simulink model "TPTC_Vehicle_dynamics_pedal2torque_NeglectSOC"  (R2026a)
settings: Solver=ode23tb  StopTime=40
model workspace (MAT data in the model file):
  BattChrgMax = -500000
  BattDischrgMax = 500000
  ChrgLmt_bpt = [1 1 1 1 1 1 1 1 0.7 0.35 0]
  DischrgLmt_bpt = [0 0.35 0.7 1 1 1 1 1 1 1 1]
  SOC_bpt = [0 10 20 30 40 50 60 70 80 90 100]
  motorMaxTorqueNm = [500 500 500 500 500 500 416.666666667 357.142857143 312.5 277.777777778 250 227.272727273 ... (16 elements, 1x16)]
  motorSpeedRadPs = [0 40 80 120 160 200 240 280 320 360 400 440 ... (16 elements, 1x16)]
values from neighbouring files (symbols this model uses):
  alpha_thr = Simulink.Parameter(300)    [init_MCU_ASR_params_only.m]
  eta_drv = Simulink.Parameter(0.95)    [init_MCU_ASR_params_only.m]
  gear_ratio_F = Simulink.Parameter(10.91)    [init_MCU_ASR_params_only.m]
  gear_ratio_R = Simulink.Parameter(11.62)    [init_MCU_ASR_params_only.m]
  J_axle = Simulink.Parameter(2*I_tire)    [init_MCU_ASR_params_only.m]
  Kd_damp = Simulink.Parameter(0.025)    [init_MCU_ASR_params_only.m]
  R_tire = Simulink.Parameter(r)    [init_MCU_ASR_params_only.m]
  T_active = Simulink.Parameter(15)    [init_MCU_ASR_params_only.m]
  T_damp_lim = Simulink.Parameter(18)    [init_MCU_ASR_params_only.m]
  tau_lpf_damp = Simulink.Parameter(0.060)    [init_MCU_ASR_params_only.m]
  Tlim_down_rate = Simulink.Parameter(2000)    [init_MCU_ASR_params_only.m]
  Tlim_up_rate = Simulink.Parameter(120)    [init_MCU_ASR_params_only.m]
  Tlim_warn_rate = Simulink.Parameter(600)    [init_MCU_ASR_params_only.m]
  Tmax_mot = Simulink.Parameter(Tn_motor)    [init_MCU_ASR_params_only.m]
  Ts_asr = Simulink.Parameter(0.001)    [init_MCU_ASR_params_only.m]
undefined symbols (not defined in the file or in its folder): dspblkCoreblockFVToolHelper, gcbh, gear_ratio
libraries: autolibsharedcoupling x8, simulink x3, autolibshareddiff x2, autolibmappedmotor x2, slpidlib x1, autolibdatasheetbattery x1, sim3dlib x1, sim3dautolib x1, vehdynlibsteering x1
(part 2 of 4)

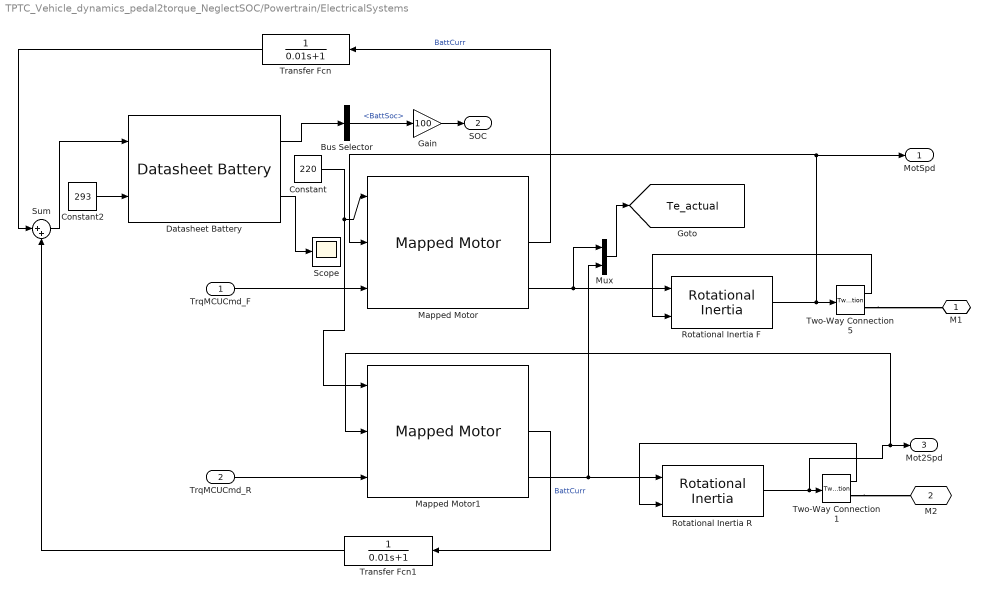
== system TPTC_Vehicle_dynamics_pedal2torque_NeglectSOC/Powertrain/ElectricalSystems ==
  TrqMCUCmd_F : Inport
  TrqMCUCmd_R : Inport  Port=2
  Bus Selector : BusSelector  OutputSignals=BattSoc
  Constant : Constant  Value=220
  Constant2 : Constant  Value=293
  Datasheet Battery : autolibdatasheetbattery/Datasheet Battery  CapacityCtrl=Parameter  OutputVlt=Unfiltered  BattChargeMax=100  Em=[2.8 3.228 3.284 3.361 3.408 3.427 3.472 3.477 3.493 3.504 3.516 3.528 3.537 3.545 3.555 3.561 3.566 3.576 3.587 3.589 3.594 3.6 3.608 3.61 3.616 3.619 3.626 3.632 3.637 3.64 3.645 3.646 3.652 3.655 3.658 3.661 3.664 3.668 3.673 3.678 3.68 3.681 3.686 3.692 3.699 3.702 3.705 3.71 3.717 3.723 3.728 3.733 3.735 3.742 3.749 3.755 3.761 3.768 3.773 3.78 3.791 3.798 3.798 3.814 3.818 3.825 3.841 3.846 3.855 3.863 3.877 3.885 3.894 3.907 3.919 3.926 3.935 3.944 3.954 3.964 3.974 3.988 3.998 4.014 4.029 4.034 4.047 4.065 4.074 4.086 4.097 4.131 4.126 4.138 4.15 4.18 4.174 4.187 4.207 4.231 4.221]  SOCEmBp=[0 0.01 0.02 0.03 0.04 0.05 0.06 0.07 0.08 0.09 0.1 0.11 0.12 0.13 0.14 0.15 0.16 0.17 0.18 0.19 0.2 0.21 0.22 0.23 0.24 0.25 0.26 0.27 0.28 0.29 0.3 0.31 0.32 0.33 0.34 0.35 0.36 0.37 0.38 0.39 0.4 0.41 0.42 0.43 0.44 0.45 0.46 0.47 0.48 0.49 0.5 0.51 0.52 0.53 0.54 0.55 0.56 0.57 0.58 0.59 0.6 0.61 0.62 0.63 0.64 0.65 0.66 0.67 0.68 0.69 0.7 0.71 0.72 0.73 0.74 0.75 0.76 0.77 0.78 0.79 0.8 0.81 0.82 0.83 0.84 0.85 0.86 0.87 0.88 0.89 0.9 0.91 0.92 0.93 0.94 0.95 0.96 0.97 0.98 0.99 1]  RInt=[0.008846 0.009319 0.009027 0.00847 0.01032 0.01314;0.006389 0.006554 0.005553 0.005525 0.006043 0.007805;0.004364 0.004101 0.00406 0.003452 0.003846 0.004517;0.002031 0.002563 0.002532 0.00246 0.002716 0.003047;0.001443 0.001825 0.001795 0.001778 0.001924 0.002234;0.0005603 0.0007192 0.0006887 0.0007557 0.0007355 0.001014;0.001028 0.001338 0.001 0.001536 0.001546 0.002789]  BattTempBp=[243.1 253.1 263.1 273.1 283.1 298.1 313.1]  SOCRintBp=[0 0.2 0.4 0.6 0.8 1]  Ns=30  Np=2  BattCapInit=60  Tc=1/1000  Vinit=4.221  RefBlkName='autolibdatasheetbattery/Datasheet Battery'
  Gain : Gain  Gain=100
  Mapped Motor : autolibmappedmotor/Mapped Motor  w_Tmax_bp_ext=w_Tmax_bp  Tmax_w_V_ext=Tmax_w_V  w_Tmin_bp_ext=w_Tmin_bp  Tmin_w_V_ext=Tmin_w_V  port_config=Speed  param_by=Tabulated torque-speed envelope  w_t=motorSpeedRadPs  T_t=motorMaxTorqueNm  torque_max=.1  power_max=30  SpreadsheetTqLimitsFileName=MotorCalibrationImportData.xlsx  Tmax_w_V=[0.09 0.09 0.09;0.08 0.08 0.08;0.07 0.07 0.07;0 0 0]  w_Tmax_bp=[ 0 375 750 800 ]  V_Tmax_bp=[500 750 900]  Tmin_w_V=[-0.09 -0.09 -0.09;-0.08 -0.08 -0.08;-0.07 -0.07 -0.07;0 0 0]  w_Tmin_bp=[ 0 375 750 800 ]  V_Tmin_bp=[500 750 900]  Tc=0.02  param_loss=Single efficiency measurement  SpreadsheetLossFileName=MotorCalibrationImportData.xlsx  SpreadsheetEffFileName=MotorCalibrationImportData.xlsx  eff=100  w_eff=375  T_eff=0.08  Piron=0  Pbase=0  w_eff_bp=[-8000 -4000 0 4000 8000]  T_eff_bp=[0 0.03 0.06 0.09]  Temp_eff_bp=[233.15 293.15 373.15]  V_eff_bp=[500 700 900]  losses_table=[1.49 1.67 2.21 3.10; 0.42 0.69 1.14 2.03; 0.06 0.24 0.78 1.68; 0.42 0.69 1.14 2.03; 1.49 1.67 2.21 3.10]  losses_table_3d=cat(3,1.05*[1.49 1.67 2.21 3.10; 0.42 0.69 1.14 2.03; 0.06 0.24 0.78 1.68; 0.42 0.69 1.14 2.03; 1.49 1.67 2.21 3.10],[1.49 1.67 2.21 3.10; 0.42 0.69 1.14 2.03; 0.06 0.24 0.78 1.68; 0.42 0.69 1.14 2.03; 1.49 1.67 2.21 3.10],1.03*[1.49 1.67 2.21 3.10; 0.42 0.69 1.14 2.03; 0.06 0.24 0.78 1.68; 0.42 0.69 1.14 2.03; 1.49 1.67 2.21 3.10])  losses_table_4d=cat(4,cat(3,[1.5645 0.441 0.063 0.441 1.5645;1.7535 0.7245 0.252 0.7245 1.7535;2.3205 1.197 0.819 1.197 2.3205;3.255 2.1315 1.764 2.1315 3.255],[1.5645 0.441 0.063 0.441 1.5645;1.7535 0.7245 0.252 0.7245 1.7535;2.3205 1.197 0.819 1.197 2.3205;3.255 2.1315 1.764 2.1315 3.255],[1.5645 0.441 0.063 0.441 1.5645;1.7535 0.7245 0.252 0.7245 1.7535;2.3205 1.197 0.819 1.197 2.3205;3.255 2.1315 1.764 2.1315 3.255]),cat(3,[1.49 0.42 0.06 0.42 1.49;1.67 0.69 0.24 0.69 1.67;2.21 1.14 0.78 1.14 2.21;3.1 2.03 1.68 2.03 3.1],[1.49 0.42 0.06 0.42 1.49;1.67 0.69 0.24 0.69 1.67;2.21 1.14 0.78 1.14 2.21;3.1 2.03 1.68 2.03 3.1],[1.49 0.42 0.06 0.42 1.49;1.67 0.69 0.24 0.69 1.67;2.21 1.14 0.78 1.14 2.21;3.1 2.03 1.68 2.03 3.1]),cat(3,[1.5347 0.4326 0.0618 0.4326 1.5347;1.7201 0.7107 0.2472 0.7107 1.7201;2.2763 1.1742 0.8034 1.1742 2.2763;3.193 2.0909 1.7304 2.0909 3.193],[1.5347 0.4326 0.0618 0.4326 1.5347;1.7201 0.7107 0.2472 0.7107 1.7201;2.2763 1.1742 0.8034 1.1742 2.2763;3.193 2.0909 1.7304 2.0909 3.193],[1.5347 0.4326 0.0618 0.4326 1.5347;1.7201 0.7107 0.2472 0.7107 1.7201;2.2763 1.1742 0.8034 1.1742 2.2763;3.193 2.0909 1.7304 2.0909 3.193]))  efficiency_table=[95 95 95 95; 95 95 95 95; 95 95 95 95; 95 95 95 95; 95 95 95 95]  efficiency_table_3d=cat(3,90*ones(5,4),95*ones(5,4),92*ones(5,4))  efficiency_table_4d=cat(4,cat(3,90*ones(5,4)',90*ones(5,4)',90*ones(5,4)'),cat(3,95*ones(5,4)',95*ones(5,4)',95*ones(5,4)'),cat(3,92*ones(5,4)',92*ones(5,4)',92*ones(5,4)'))  J=5e-6  b=1e-5  omega_o=0  T_t_extended=[166.666666666667 178.571428571429 192.307692307692 208.333333333333 227.272727272727 250 277.777777777778 312.5 357.142857142857 416.666666666667 500 500 500 500 500 500 500 500 500 500 500 416.666666666667 357.142857142857 312.5 277.777777777778 250 227.272727272727 208.333333333333 192.307692307692 178.571428571429 166.666666666667]  w_t_extended=[-600 -560 -520 -480 -440 -400 -360 -320 -280 -240 -200 -160 -120 -80 -40 0 40 80 120 160 200 240 280 320 360 400 440 480 520 560 600]  KLossIron=0  KLossCopper=0  x_w_eff_vec=[-8000 -4000 0 4000 8000]  x_T_eff_vec=[-0.09 -0.06 -0.03 0 0.03 0.06 0.09]  x_tmp_eff_vec=[233.15 293.15 373.15]  x_V_eff_vec=[500 700 900]  x_losses_mat=[3.1 2.21 1.67 1.49 1.67 2.21 3.1;2.03 1.14 0.69 0.42 0.69 1.14 2.03;1.68 0.78 0.24 0.06 0.24 0.78 1.68;2.03 1.14 0.69 0.42 0.69 1.14 2.03;3.1 2.21 1.67 1.49 1.67 2.21 3.1]  x_losses_mat_3d=cat(3,[3.255 2.3205 1.7535 1.5645 1.7535 2.3205 3.255;2.1315 1.197 0.7245 0.441 0.7245 1.197 2.1315;1.764 0.819 0.252 0.063 0.252 0.819 1.764;2.1315 1.197 0.7245 0.441 0.7245 1.197 2.1315;3.255 2.3205 1.7535 1.5645 1.7535 2.3205 3.255],[3.1 2.21 1.67 1.49 1.67 2.21 3.1;2.03 1.14 0.69 0.42 0.69 1.14 2.03;1.68 0.78 0.24 0.06 0.24 0.78 1.68;2.03 1.14 0.69 0.42 0.69 1.14 2.03;3.1 2.21 1.67 1.49 1.67 2.21 3.1],[3.193 2.2763 1.7201 1.5347 1.7201 2.2763 3.193;2.0909 1.1742 0.7107 0.4326 0.7107 1.1742 2.0909;1.7304 0.8034 0.2472 0.0618 0.2472 0.8034 1.7304;2.0909 1.1742 0.7107 0.4326 0.7107 1.1742 2.0909;3.193 2.2763 1.7201 1.5347 1.7201 2.2763 3.193])  x_losses_mat_4d=cat(4,cat(3,[1.5645 0.441 0.063 0.441 1.5645;1.7535 0.7245 0.252 0.7245 1.7535;2.3205 1.197 0.819 1.197 2.3205;3.255 2.1315 1.764 2.1315 3.255],[1.5645 0.441 0.063 0.441 1.5645;1.7535 0.7245 0.252 0.7245 1.7535;2.3205 1.197 0.819 1.197 2.3205;3.255 2.1315 1.764 2.1315 3.255],[1.5645 0.441 0.063 0.441 1.5645;1.7535 0.7245 0.252 0.7245 1.7535;2.3205 1.197 0.819 1.197 2.3205;3.255 2.1315 1.764 2.1315 3.255]),cat(3,[1.49 0.42 0.06 0.42 1.49;1.67 0.69 0.24 0.69 1.67;2.21 1.14 0.78 1.14 2.21;3.1 2.03 1.68 2.03 3.1],[1.49 0.42 0.06 0.42 1.49;1.67 0.69 0.24 0.69 1.67;2.21 1.14 0.78 1.14 2.21;3.1 2.03 1.68 2.03 3.1],[1.49 0.42 0.06 0.42 1.49;1.67 0.69 0.24 0.69 1.67;2.21 1.14 0.78 1.14 2.21;3.1 2.03 1.68 2.03 3.1]),cat(3,[1.5347 0.4326 0.0618 0.4326 1.5347;1.7201 0.7107 0.2472 0.7107 1.7201;2.2763 1.1742 0.8034 1.1742 2.2763;3.193 2.0909 1.7304 2.0909 3.193],[1.5347 0.4326 0.0618 0.4326 1.5347;1.7201 0.7107 0.2472 0.7107 1.7201;2.2763 1.1742 0.8034 1.1742 2.2763;3.193 2.0909 1.7304 2.0909 3.193],[1.5347 0.4326 0.0618 0.4326 1.5347;1.7201 0.7107 0.2472 0.7107 1.7201;2.2763 1.1742 0.8034 1.1742 2.2763;3.193 2.0909 1.7304 2.0909 3.193]))  CalLossMapData={}  CalLossWithTempMapData={}  aMode=aMode  RefBlkName='autolibmappedmotor/Mapped Motor'
  Mapped Motor1 : autolibmappedmotor/Mapped Motor  w_Tmax_bp_ext=w_Tmax_bp  Tmax_w_V_ext=Tmax_w_V  w_Tmin_bp_ext=w_Tmin_bp  Tmin_w_V_ext=Tmin_w_V  port_config=Speed  param_by=Tabulated torque-speed envelope  w_t=motorSpeedRadPs  T_t=motorMaxTorqueNm  torque_max=.1  power_max=30  SpreadsheetTqLimitsFileName=MotorCalibrationImportData.xlsx  Tmax_w_V=[0.09 0.09 0.09;0.08 0.08 0.08;0.07 0.07 0.07;0 0 0]  w_Tmax_bp=[ 0 375 750 800 ]  V_Tmax_bp=[500 750 900]  Tmin_w_V=[-0.09 -0.09 -0.09;-0.08 -0.08 -0.08;-0.07 -0.07 -0.07;0 0 0]  w_Tmin_bp=[ 0 375 750 800 ]  V_Tmin_bp=[500 750 900]  Tc=0.02  param_loss=Single efficiency measurement  SpreadsheetLossFileName=MotorCalibrationImportData.xlsx  SpreadsheetEffFileName=MotorCalibrationImportData.xlsx  eff=100  w_eff=375  T_eff=0.08  Piron=0  Pbase=0  w_eff_bp=[-8000 -4000 0 4000 8000]  T_eff_bp=[0 0.03 0.06 0.09]  Temp_eff_bp=[233.15 293.15 373.15]  V_eff_bp=[500 700 900]  losses_table=[1.49 1.67 2.21 3.10; 0.42 0.69 1.14 2.03; 0.06 0.24 0.78 1.68; 0.42 0.69 1.14 2.03; 1.49 1.67 2.21 3.10]  losses_table_3d=cat(3,1.05*[1.49 1.67 2.21 3.10; 0.42 0.69 1.14 2.03; 0.06 0.24 0.78 1.68; 0.42 0.69 1.14 2.03; 1.49 1.67 2.21 3.10],[1.49 1.67 2.21 3.10; 0.42 0.69 1.14 2.03; 0.06 0.24 0.78 1.68; 0.42 0.69 1.14 2.03; 1.49 1.67 2.21 3.10],1.03*[1.49 1.67 2.21 3.10; 0.42 0.69 1.14 2.03; 0.06 0.24 0.78 1.68; 0.42 0.69 1.14 2.03; 1.49 1.67 2.21 3.10])  losses_table_4d=cat(4,cat(3,[1.5645 0.441 0.063 0.441 1.5645;1.7535 0.7245 0.252 0.7245 1.7535;2.3205 1.197 0.819 1.197 2.3205;3.255 2.1315 1.764 2.1315 3.255],[1.5645 0.441 0.063 0.441 1.5645;1.7535 0.7245 0.252 0.7245 1.7535;2.3205 1.197 0.819 1.197 2.3205;3.255 2.1315 1.764 2.1315 3.255],[1.5645 0.441 0.063 0.441 1.5645;1.7535 0.7245 0.252 0.7245 1.7535;2.3205 1.197 0.819 1.197 2.3205;3.255 2.1315 1.764 2.1315 3.255]),cat(3,[1.49 0.42 0.06 0.42 1.49;1.67 0.69 0.24 0.69 1.67;2.21 1.14 0.78 1.14 2.21;3.1 2.03 1.68 2.03 3.1],[1.49 0.42 0.06 0.42 1.49;1.67 0.69 0.24 0.69 1.67;2.21 1.14 0.78 1.14 2.21;3.1 2.03 1.68 2.03 3.1],[1.49 0.42 0.06 0.42 1.49;1.67 0.69 0.24 0.69 1.67;2.21 1.14 0.78 1.14 2.21;3.1 2.03 1.68 2.03 3.1]),cat(3,[1.5347 0.4326 0.0618 0.4326 1.5347;1.7201 0.7107 0.2472 0.7107 1.7201;2.2763 1.1742 0.8034 1.1742 2.2763;3.193 2.0909 1.7304 2.0909 3.193],[1.5347 0.4326 0.0618 0.4326 1.5347;1.7201 0.7107 0.2472 0.7107 1.7201;2.2763 1.1742 0.8034 1.1742 2.2763;3.193 2.0909 1.7304 2.0909 3.193],[1.5347 0.4326 0.0618 0.4326 1.5347;1.7201 0.7107 0.2472 0.7107 1.7201;2.2763 1.1742 0.8034 1.1742 2.2763;3.193 2.0909 1.7304 2.0909 3.193]))  efficiency_table=[95 95 95 95; 95 95 95 95; 95 95 95 95; 95 95 95 95; 95 95 95 95]  efficiency_table_3d=cat(3,90*ones(5,4),95*ones(5,4),92*ones(5,4))  efficiency_table_4d=cat(4,cat(3,90*ones(5,4)',90*ones(5,4)',90*ones(5,4)'),cat(3,95*ones(5,4)',95*ones(5,4)',95*ones(5,4)'),cat(3,92*ones(5,4)',92*ones(5,4)',92*ones(5,4)'))  J=5e-6  b=1e-5  omega_o=0  T_t_extended=[166.666666666667 178.571428571429 192.307692307692 208.333333333333 227.272727272727 250 277.777777777778 312.5 357.142857142857 416.666666666667 500 500 500 500 500 500 500 500 500 500 500 416.666666666667 357.142857142857 312.5 277.777777777778 250 227.272727272727 208.333333333333 192.307692307692 178.571428571429 166.666666666667]  w_t_extended=[-600 -560 -520 -480 -440 -400 -360 -320 -280 -240 -200 -160 -120 -80 -40 0 40 80 120 160 200 240 280 320 360 400 440 480 520 560 600]  KLossIron=0  KLossCopper=0  x_w_eff_vec=[-8000 -4000 0 4000 8000]  x_T_eff_vec=[-0.09 -0.06 -0.03 0 0.03 0.06 0.09]  x_tmp_eff_vec=[233.15 293.15 373.15]  x_V_eff_vec=[500 700 900]  x_losses_mat=[3.1 2.21 1.67 1.49 1.67 2.21 3.1;2.03 1.14 0.69 0.42 0.69 1.14 2.03;1.68 0.78 0.24 0.06 0.24 0.78 1.68;2.03 1.14 0.69 0.42 0.69 1.14 2.03;3.1 2.21 1.67 1.49 1.67 2.21 3.1]  x_losses_mat_3d=cat(3,[3.255 2.3205 1.7535 1.5645 1.7535 2.3205 3.255;2.1315 1.197 0.7245 0.441 0.7245 1.197 2.1315;1.764 0.819 0.252 0.063 0.252 0.819 1.764;2.1315 1.197 0.7245 0.441 0.7245 1.197 2.1315;3.255 2.3205 1.7535 1.5645 1.7535 2.3205 3.255],[3.1 2.21 1.67 1.49 1.67 2.21 3.1;2.03 1.14 0.69 0.42 0.69 1.14 2.03;1.68 0.78 0.24 0.06 0.24 0.78 1.68;2.03 1.14 0.69 0.42 0.69 1.14 2.03;3.1 2.21 1.67 1.49 1.67 2.21 3.1],[3.193 2.2763 1.7201 1.5347 1.7201 2.2763 3.193;2.0909 1.1742 0.7107 0.4326 0.7107 1.1742 2.0909;1.7304 0.8034 0.2472 0.0618 0.2472 0.8034 1.7304;2.0909 1.1742 0.7107 0.4326 0.7107 1.1742 2.0909;3.193 2.2763 1.7201 1.5347 1.7201 2.2763 3.193])  x_losses_mat_4d=cat(4,cat(3,[1.5645 0.441 0.063 0.441 1.5645;1.7535 0.7245 0.252 0.7245 1.7535;2.3205 1.197 0.819 1.197 2.3205;3.255 2.1315 1.764 2.1315 3.255],[1.5645 0.441 0.063 0.441 1.5645;1.7535 0.7245 0.252 0.7245 1.7535;2.3205 1.197 0.819 1.197 2.3205;3.255 2.1315 1.764 2.1315 3.255],[1.5645 0.441 0.063 0.441 1.5645;1.7535 0.7245 0.252 0.7245 1.7535;2.3205 1.197 0.819 1.197 2.3205;3.255 2.1315 1.764 2.1315 3.255]),cat(3,[1.49 0.42 0.06 0.42 1.49;1.67 0.69 0.24 0.69 1.67;2.21 1.14 0.78 1.14 2.21;3.1 2.03 1.68 2.03 3.1],[1.49 0.42 0.06 0.42 1.49;1.67 0.69 0.24 0.69 1.67;2.21 1.14 0.78 1.14 2.21;3.1 2.03 1.68 2.03 3.1],[1.49 0.42 0.06 0.42 1.49;1.67 0.69 0.24 0.69 1.67;2.21 1.14 0.78 1.14 2.21;3.1 2.03 1.68 2.03 3.1]),cat(3,[1.5347 0.4326 0.0618 0.4326 1.5347;1.7201 0.7107 0.2472 0.7107 1.7201;2.2763 1.1742 0.8034 1.1742 2.2763;3.193 2.0909 1.7304 2.0909 3.193],[1.5347 0.4326 0.0618 0.4326 1.5347;1.7201 0.7107 0.2472 0.7107 1.7201;2.2763 1.1742 0.8034 1.1742 2.2763;3.193 2.0909 1.7304 2.0909 3.193],[1.5347 0.4326 0.0618 0.4326 1.5347;1.7201 0.7107 0.2472 0.7107 1.7201;2.2763 1.1742 0.8034 1.1742 2.2763;3.193 2.0909 1.7304 2.0909 3.193]))  CalLossMapData={}  CalLossWithTempMapData={}  aMode=aMode  RefBlkName='autolibmappedmotor/Mapped Motor'
  Mux : Mux  Inputs=2
  Rotational Inertia F : autolibsharedcoupling/Rotational Inertia  port_config=Simulink  extInfo=off  externJ=off  J=.001  b=.001  omega_o=0  blkID=0  aMode=1
      settings: LibrarySourceBlock=autolibcoupling/Rotational Inertia
  Rotational Inertia R : autolibsharedcoupling/Rotational Inertia  port_config=Simulink  extInfo=off  externJ=off  J=.001  b=.001  omega_o=0  blkID=0  aMode=1
      settings: LibrarySourceBlock=autolibcoupling/Rotational Inertia
  Scope : Scope
      settings: ActiveDisplayYMinimum=56.73874  ActiveDisplayYMaximum=120.06236  DataLoggingVariableName=ScopeData18
  Sum : Sum  Inputs=|++
  Transfer Fcn : TransferFcn  Denominator=[0.01 1]
  Transfer Fcn1 : TransferFcn  Denominator=[0.01 1]
  Two-Way Connection1 : TwoWayConnection
  Two-Way Connection5 : TwoWayConnection
  M1 : PMIOPort  Side=Right
  M2 : PMIOPort  Port=2  Side=Right
  MotSpd : Outport
  SOC : Outport  Port=2
  Mot2Spd : Outport  Port=3
  tag scope: Te_actual=global
  wires:
  Rotational Inertia F/1 -> Mapped Motor/2, MotSpd/1, Two-Way Connection5/1
  Datasheet Battery/2 -> Scope/1
  Mapped Motor/3 -> Mux/1, Rotational Inertia F/1
  TrqMCUCmd_F/1 -> Mapped Motor/3
  Two-Way Connection5/1 -> Rotational Inertia F/2
  Constant2/1 -> Datasheet Battery/2
  Mapped Motor/2 -> Transfer Fcn/1  "BattCurr"
  Datasheet Battery/1 -> Bus Selector/1
  Bus Selector/1 -> Gain/1  "<BattSoc>"
  Gain/1 -> SOC/1
  Rotational Inertia R/1 -> Mapped Motor1/2, Mot2Spd/1, Two-Way Connection1/1
  Mapped Motor1/3 -> Mux/2, Rotational Inertia R/1
  Two-Way Connection1/1 -> Rotational Inertia R/2
  TrqMCUCmd_R/1 -> Mapped Motor1/3
  Mapped Motor1/2 -> Transfer Fcn1/1  "BattCurr"
  Transfer Fcn/1 -> Sum/1
  Transfer Fcn1/1 -> Sum/2
  Sum/1 -> Datasheet Battery/1
  Mux/1 -> [Te_actual]
  Constant/1 -> Mapped Motor1/1, Mapped Motor/1
  connections:
  Two-Way Connection5/RConn1 -- M1/RConn1
  Two-Way Connection1/RConn1 -- M2/RConn1

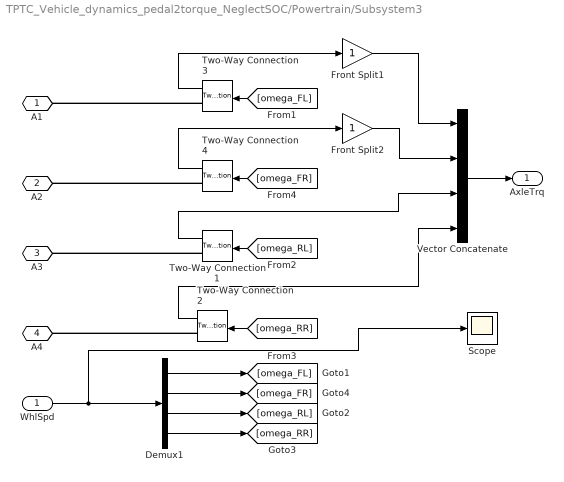
== system TPTC_Vehicle_dynamics_pedal2torque_NeglectSOC/Powertrain/Subsystem3 ==
  WhlSpd : Inport
  Demux1 : Demux
  Front Split1 : Gain
  Front Split2 : Gain
  Scope : Scope
      settings: ActiveDisplayYMinimum=-39.72739  ActiveDisplayYMaximum=357.54646  DataLoggingVariableName=ScopeData19
  Two-Way Connection{1..4} (4 alike) : TwoWayConnection
  Vector Concatenate : Concatenate  NumInputs=4
  A1 : PMIOPort  Side=Left
  A2 : PMIOPort  Port=2  Side=Left
  A3 : PMIOPort  Port=3  Side=Left
  A4 : PMIOPort  Port=4  Side=Left
  AxleTrq : Outport  VectorParamsAs1DForOutWhenUnconnected=off
  wires:
  Two-Way Connection1/1 -> Vector Concatenate/3
  Front Split1/1 -> Vector Concatenate/1
  [omega_RL] -> Two-Way Connection1/1
  Demux1/4 -> [omega_RR]
  Demux1/1 -> [omega_FL]
  Demux1/2 -> [omega_FR]
  Vector Concatenate/1 -> AxleTrq/1
  Demux1/3 -> [omega_RL]
  [omega_FL] -> Two-Way Connection3/1
  [omega_FR] -> Two-Way Connection4/1
  Front Split2/1 -> Vector Concatenate/2
  [omega_RR] -> Two-Way Connection2/1
  Two-Way Connection3/1 -> Front Split1/1
  Two-Way Connection2/1 -> Vector Concatenate/4
  WhlSpd/1 -> Scope/1, Demux1/1
  Two-Way Connection4/1 -> Front Split2/1
  connections:
  Two-Way Connection3/RConn1 -- A1/RConn1
  Two-Way Connection2/RConn1 -- A4/RConn1
  Two-Way Connection1/RConn1 -- A3/RConn1
  Two-Way Connection4/RConn1 -- A2/RConn1

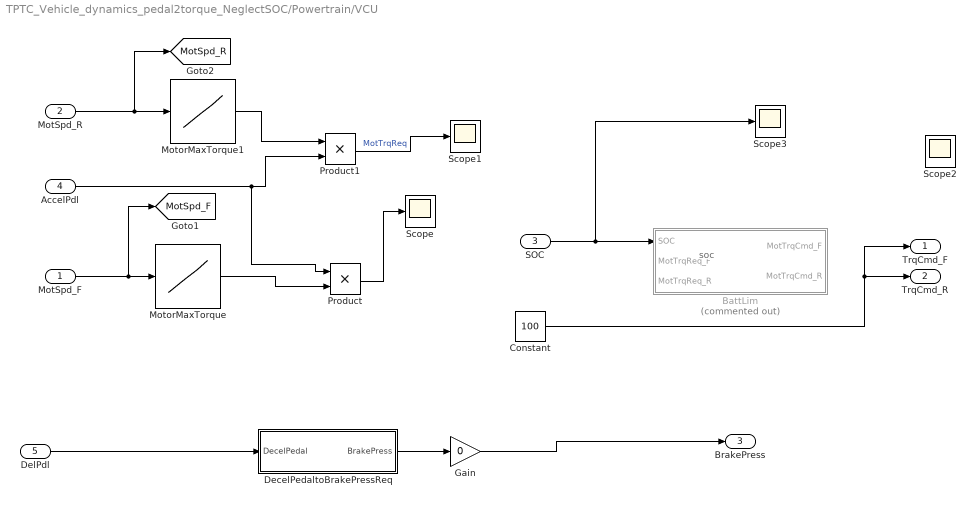
== system TPTC_Vehicle_dynamics_pedal2torque_NeglectSOC/Powertrain/VCU ==
  note: soc
  MotSpd_F : Inport
  MotSpd_R : Inport  Port=2
  SOC : Inport  Port=3
  AccelPdl : Inport  Port=4
  DelPdl : Inport  Port=5
  BattLim : Subsystem  Commented=on
  Constant : Constant  Value=100
  DecelPedaltoBrakePressReq : Subsystem
  Gain : Gain  Gain=0
  MotorMaxTorque : Lookup_n-D  NumberOfTableDimensions=1  BreakpointsForDimension1=motorSpeedRadPs  Table=motorMaxTorqueNm  ExtrapMethod=Clip  InternalRulePriority=Speed  RndMeth=Simplest
  MotorMaxTorque1 : Lookup_n-D  NumberOfTableDimensions=1  BreakpointsForDimension1=motorSpeedRadPs  Table=motorMaxTorqueNm  ExtrapMethod=Clip  InternalRulePriority=Speed  RndMeth=Simplest
  Product : Product
  Product1 : Product
  Scope{,1..3} (4 alike) : Scope
      Scope settings: ActiveDisplayYMinimum=-49.01156  ActiveDisplayYMaximum=441.10403  DataLoggingVariableName=ScopeData3
      Scope1 settings: ActiveDisplayYMinimum=-47.85141  ActiveDisplayYMaximum=430.66269  DataLoggingVariableName=ScopeData4
      Scope2 settings: ActiveDisplayYMinimum=-1  ActiveDisplayYMaximum=1  DataLoggingVariableName=ScopeData5
      Scope3 settings: ActiveDisplayYMinimum=53.4768  ActiveDisplayYMaximum=60.7248  DataLoggingVariableName=ScopeData14
  TrqCmd_F : Outport
  TrqCmd_R : Outport  Port=2
  BrakePress : Outport  Port=3
  tag scope: MotSpd_F=global, MotSpd_R=global
  wires:
  DelPdl/1 -> DecelPedaltoBrakePressReq/1(DecelPedal)
  Product/1 -> Scope/1
  MotSpd_F/1 -> MotorMaxTorque/1, [MotSpd_F]
  SOC/1 -> Scope3/1, BattLim/1(SOC)
  DecelPedaltoBrakePressReq/1(BrakePress) -> Gain/1
  MotSpd_R/1 -> [MotSpd_R], MotorMaxTorque1/1
  MotorMaxTorque1/1 -> Product1/1
  Gain/1 -> BrakePress/1
  AccelPdl/1 -> Product/1, Product1/2
  Product1/1 -> Scope1/1  "MotTrqReq"
  MotorMaxTorque/1 -> Product/2
  Constant/1 -> TrqCmd_R/1, TrqCmd_F/1

== system TPTC_Vehicle_dynamics_pedal2torque_NeglectSOC/Environment/Ground Feedback/Constant ==
  Friction : Inport
  Bus Creator : BusCreator  Inputs=4
  Bus Creator2 : BusCreator  Inputs=4
  Bus Creator3 : BusCreator  Inputs=3
  Constant1 : Constant  Value=zeros(4,1)
  Constant2 : Constant  Value=repmat(eye(3),1,1,4)  SampleTime=-1
  Demux : Demux
  Demux1 : Demux
  Signal Specification : SignalSpecification  Unit=m
  Signal Specification1 : SignalSpecification  Unit=1
  Ground : Outport  VectorParamsAs1DForOutWhenUnconnected=off
  wires:
  Constant1/1 -> Signal Specification/1
  Signal Specification/1 -> Demux/1
  Demux/4 -> Bus Creator/4  "G_RR_z"
  Demux/1 -> Bus Creator/1  "G_FL_z"
  Demux/3 -> Bus Creator/3  "G_RL_z"
  Demux/2 -> Bus Creator/2  "G_FR_z"
  Bus Creator/1 -> Bus Creator3/1  "z"
  Demux1/3 -> Bus Creator2/3  "mu_RL"
  Demux1/4 -> Bus Creator2/4  "mu_RR"
  Demux1/1 -> Bus Creator2/1  "mu_FL"
  Demux1/2 -> Bus Creator2/2  "mu_FR"
  Bus Creator2/1 -> Bus Creator3/3  "mu"
  Friction/1 -> Signal Specification1/1
  Signal Specification1/1 -> Demux1/1
  Bus Creator3/1 -> Ground/1
  Constant2/1 -> Bus Creator3/2  "DCM"

== system TPTC_Vehicle_dynamics_pedal2torque_NeglectSOC/Powertrain/03_MCU_TPTC_Controller/Command_Merge_Front ==
  T_vcu : Inport
  Tlim : Inport  Port=2
  T_damp : Inport  Port=3
  Demux1 : Demux  Outputs=2
  Demux2 : Demux  Outputs=2
  Demux3 : Demux  Outputs=2
  Fast_Down_Slow_Up_Limiter : MATLAB Function  TreatAsAtomicUnit=on
  Scope : Scope  NumInputPorts=3
      settings: ActiveDisplayYMinimum=99.91686  ActiveDisplayYMaximum=100.00924  DataLoggingVariableName=ScopeData13
  MT_vcu_f : Outport
  MT_vcu_r : Outport  Port=2
  wires:
  Fast_Down_Slow_Up_Limiter/2(T_cmd_r) -> Scope/2, MT_vcu_r/1
  Fast_Down_Slow_Up_Limiter/1(T_cmd_f) -> Scope/1, MT_vcu_f/1
  Demux1/1 -> Fast_Down_Slow_Up_Limiter/1(T_vcu_f)
  Demux1/2 -> Fast_Down_Slow_Up_Limiter/2(T_vcu_r)
  Tlim/1 -> Demux2/1
  Demux2/1 -> Fast_Down_Slow_Up_Limiter/3(Tlim_f)
  Demux2/2 -> Fast_Down_Slow_Up_Limiter/4(Tlim_r)
  T_damp/1 -> Demux3/1
  Demux3/1 -> Fast_Down_Slow_Up_Limiter/5(T_damp_f)
  Demux3/2 -> Fast_Down_Slow_Up_Limiter/6(T_damp_r)
  T_vcu/1 -> Scope/3, Demux1/1

== system TPTC_Vehicle_dynamics_pedal2torque_NeglectSOC/Powertrain/03_MCU_TPTC_Controller/Load_Observer ==
  Te_hat_F : Inport
  alpha_motor_F : Inport  Port=2
  Te_hat_R : Inport  Port=3
  alpha_motor_R : Inport  Port=4
  J_eq_motor : Gain  Gain=J_axle
  J_eq_motor1 : Gain  Gain=J_axle
  Saturation_nonnegative : Saturate  UpperLimit=Tmax_mot  LowerLimit=0
  Saturation_nonnegative1 : Saturate  UpperLimit=Tmax_mot  LowerLimit=0
  Scope1 : Scope
      settings: ActiveDisplayYMinimum=-88.64455  ActiveDisplayYMaximum=794.81375  DataLoggingVariableName=ScopeData13
  Scope2 : Scope
      settings: ActiveDisplayYMinimum=-126.82581  ActiveDisplayYMaximum=95.18241  DataLoggingVariableName=ScopeData14
  Scope3 : Scope
      settings: ActiveDisplayYMinimum=-4613.8951  ActiveDisplayYMaximum=4308.81674  DataLoggingVariableName=ScopeData16
  Te_minus_Jalpha : Sum  Inputs=+-
  Te_minus_Jalpha1 : Sum  Inputs=+-
  Tload_hat_F : Outport
  Tload_hat_R : Outport  Port=2
  wires:
  alpha_motor_F/1 -> Scope3/1, J_eq_motor/1
  Te_hat_F/1 -> Te_minus_Jalpha/1
  J_eq_motor/1 -> Scope2/1, Te_minus_Jalpha/2
  Te_minus_Jalpha/1 -> Scope1/1, Saturation_nonnegative/1
  Saturation_nonnegative/1 -> Tload_hat_F/1
  Te_hat_R/1 -> Te_minus_Jalpha1/1
  Saturation_nonnegative1/1 -> Tload_hat_R/1
  J_eq_motor1/1 -> Te_minus_Jalpha1/2
  alpha_motor_R/1 -> J_eq_motor1/1
  Te_minus_Jalpha1/1 -> Saturation_nonnegative1/1

== system TPTC_Vehicle_dynamics_pedal2torque_NeglectSOC/Powertrain/03_MCU_TPTC_Controller/Motor_Acceleration_Estimation ==
  omega_m_f : Inport
  omega_m_r : Inport  Port=2
  Discrete Transfer Fcn : DiscreteTransferFcn  LoadFcn=dspblkCoreblockFVToolHelper(gcbh,'load');  Numerator=[0.0487706]  Denominator=[1 -0.951229]
      settings: CopyFcn=dspblkCoreblockFVToolHelper(gcbh,'copy');  DeleteFcn=dspblkCoreblockFVToolHelper(gcbh,'close');  ModelCloseFcn=dspblkCoreblockFVToolHelper(gcbh,'close');  PreSaveFcn=dspblkCoreblockFVToolHelper(gcbh,'presave');  PostSaveFcn=dspblkCoreblockFVToolHelper(gcbh,'postsave');  CloseFcn=dspblkCoreblockFVToolHelper(gcbh,'close');
  Discrete Transfer Fcn1 : DiscreteTransferFcn  LoadFcn=dspblkCoreblockFVToolHelper(gcbh,'load');  Numerator=[0.0487706]  Denominator=[1 -0.951229]
      settings: CopyFcn=dspblkCoreblockFVToolHelper(gcbh,'copy');  DeleteFcn=dspblkCoreblockFVToolHelper(gcbh,'close');  ModelCloseFcn=dspblkCoreblockFVToolHelper(gcbh,'close');  PreSaveFcn=dspblkCoreblockFVToolHelper(gcbh,'presave');  PostSaveFcn=dspblkCoreblockFVToolHelper(gcbh,'postsave');  CloseFcn=dspblkCoreblockFVToolHelper(gcbh,'close');
  Gain : Gain  Gain=1/Ts_asr
  Gain1 : Gain  Gain=1/Ts_asr
  Sum : Sum  Inputs=|+-
  Sum1 : Sum  Inputs=|+-
  Unit Delay : UnitDelay  SampleTime=-1
  Unit Delay1 : UnitDelay  SampleTime=-1
  alpha_m_f : Outport
  alpha_m_r : Outport  Port=2
  wires:
  omega_m_f/1 -> Sum/1, Unit Delay/1
  Unit Delay/1 -> Sum/2
  Sum/1 -> Gain/1
  Gain/1 -> Discrete Transfer Fcn/1
  Discrete Transfer Fcn/1 -> alpha_m_f/1
  Gain1/1 -> Discrete Transfer Fcn1/1
  omega_m_r/1 -> Sum1/1, Unit Delay1/1
  Sum1/1 -> Gain1/1
  Unit Delay1/1 -> Sum1/2
  Discrete Transfer Fcn1/1 -> alpha_m_r/1

== system TPTC_Vehicle_dynamics_pedal2torque_NeglectSOC/Powertrain/03_MCU_TPTC_Controller/ReaL_Load_Force ==
  Add1 : Sum
  Add2 : Sum
  Demux : Demux
  Demux1 : Demux
  F to Torque : Gain  Gain=R_tire *1 / (gear_ratio_R * eta_drv);
  F to Torque1 : Gain  Gain=R_tire *1 / (gear_ratio_F * eta_drv);
  ReaL_Load_Force_Front : Outport
  ReaL_Load_Force_Rear : Outport  Port=2
  wires:
  Demux1/2 -> Add2/2
  F to Torque/1 -> Demux/1
  [Fx] -> F to Torque1/1
  [Fx] -> F to Torque/1
  F to Torque1/1 -> Demux1/1
  Demux/4 -> Add1/2
  Demux/3 -> Add1/1
  Demux1/1 -> Add2/1
  Add2/1 -> ReaL_Load_Force_Front/1
  Add1/1 -> ReaL_Load_Force_Rear/1

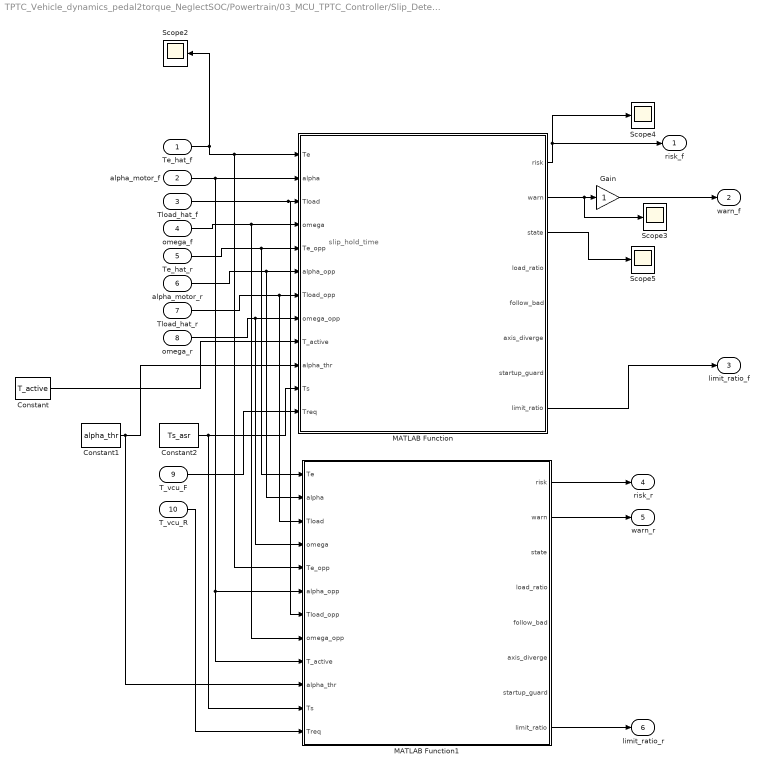
== system TPTC_Vehicle_dynamics_pedal2torque_NeglectSOC/Powertrain/03_MCU_TPTC_Controller/Slip_Detector_Front ==
  note: slip_hold_time
  Te_hat_f : Inport
  alpha_motor_f : Inport  Port=2
  Tload_hat_f : Inport  Port=3
  omega_f : Inport  Port=4
  Te_hat_r : Inport  Port=5
  alpha_motor_r : Inport  Port=6
  Tload_hat_r : Inport  Port=7
  omega_r : Inport  Port=8
  T_vcu_F : Inport  Port=9
  T_vcu_R : Inport  Port=10
  Constant : Constant  Value=T_active
  Constant1 : Constant  Value=alpha_thr
  Constant2 : Constant  Value=Ts_asr
  Gain : Gain
  MATLAB Function : MATLAB Function  TreatAsAtomicUnit=on  SystemSampleTime=Ts_asr
  MATLAB Function1 : MATLAB Function  TreatAsAtomicUnit=on  SystemSampleTime=Ts_asr
  Scope{2..5} (4 alike) : Scope
      Scope2 settings: ActiveDisplayYMinimum=-72.34212  ActiveDisplayYMaximum=651.07911  DataLoggingVariableName=ScopeData11
      Scope3 settings: ActiveDisplayYMinimum=-1  ActiveDisplayYMaximum=1  DataLoggingVariableName=ScopeData12
      Scope4 settings: ActiveDisplayYMinimum=-1  ActiveDisplayYMaximum=1  DataLoggingVariableName=ScopeData9
      Scope5 settings: ActiveDisplayYMinimum=-0.24999999999999994  ActiveDisplayYMaximum=2.25
  risk_f : Outport
  warn_f : Outport  Port=2
  limit_ratio_f : Outport  Port=3
  risk_r : Outport  Port=4
  warn_r : Outport  Port=5
  limit_ratio_r : Outport  Port=6
  wires:
  Tload_hat_f/1 -> MATLAB Function1/7(Tload_opp), MATLAB Function/3(Tload)
  alpha_motor_f/1 -> MATLAB Function1/9(T_active), MATLAB Function1/6(alpha_opp), MATLAB Function/2(alpha)
  Te_hat_f/1 -> Scope2/1, MATLAB Function1/5(Te_opp), MATLAB Function/1(Te)
  MATLAB Function/1(risk) -> Scope4/1, risk_f/1
  MATLAB Function/2(warn) -> Scope3/1, Gain/1
  MATLAB Function/3(state) -> Scope5/1
  Gain/1 -> warn_f/1
  omega_f/1 -> MATLAB Function1/8(omega_opp), MATLAB Function/4(omega)
  alpha_motor_r/1 -> MATLAB Function1/2(alpha), MATLAB Function/6(alpha_opp)
  Tload_hat_r/1 -> MATLAB Function1/3(Tload), MATLAB Function/7(Tload_opp)
  omega_r/1 -> MATLAB Function1/4(omega), MATLAB Function/8(omega_opp)
  Constant/1 -> MATLAB Function/9(T_active)
  Constant1/1 -> MATLAB Function/10(alpha_thr), MATLAB Function1/10(alpha_thr)
  Constant2/1 -> MATLAB Function1/11(Ts), MATLAB Function/11(Ts)
  T_vcu_F/1 -> MATLAB Function/12(Treq)
  MATLAB Function/8(limit_ratio) -> limit_ratio_f/1
  Te_hat_r/1 -> MATLAB Function1/1(Te), MATLAB Function/5(Te_opp)
  MATLAB Function1/8(limit_ratio) -> limit_ratio_r/1
  MATLAB Function1/1(risk) -> risk_r/1
  MATLAB Function1/2(warn) -> warn_r/1
  T_vcu_R/1 -> MATLAB Function1/12(Treq)

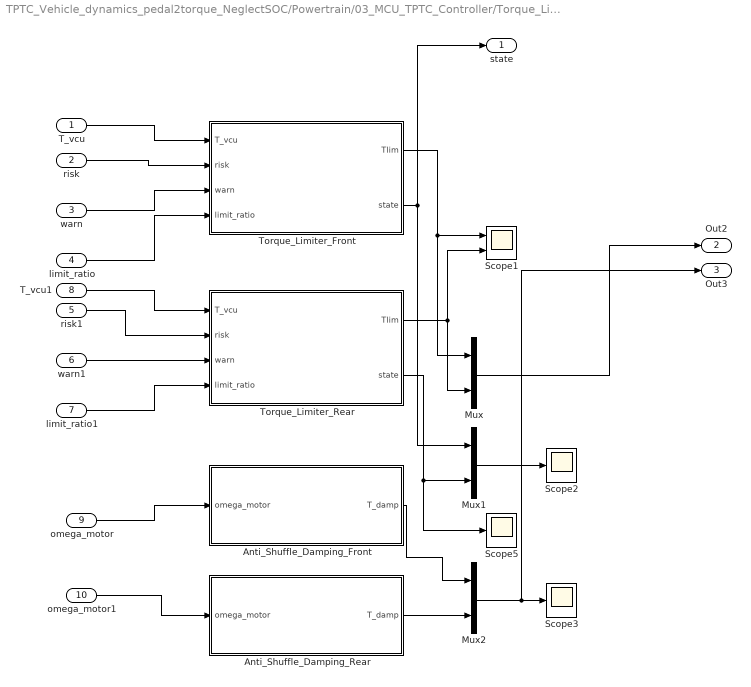
== system TPTC_Vehicle_dynamics_pedal2torque_NeglectSOC/Powertrain/03_MCU_TPTC_Controller/Torque_Limiter ==
  T_vcu : Inport
  risk : Inport  Port=2
  warn : Inport  Port=3
  limit_ratio : Inport  Port=4
  risk1 : Inport  Port=5
  warn1 : Inport  Port=6
  limit_ratio1 : Inport  Port=7
  T_vcu1 : Inport  Port=8
  omega_motor : Inport  Port=9
  omega_motor1 : Inport  Port=10
  Anti_Shuffle_Damping_Front : Subsystem
  Anti_Shuffle_Damping_Rear : Subsystem
  Mux : Mux  Inputs=2
  Mux1 : Mux  Inputs=2
  Mux2 : Mux  Inputs=2
  Scope1 : Scope  NumInputPorts=2
      settings: ActiveDisplayYMinimum=90  ActiveDisplayYMaximum=110  DataLoggingVariableName=ScopeData7
  Scope2 : Scope
      settings: ActiveDisplayYMinimum=-0.12499999999999997  ActiveDisplayYMaximum=1.125
  Scope3 : Scope
      settings: ActiveDisplayYMinimum=-1  ActiveDisplayYMaximum=1  DataLoggingVariableName=ScopeData8
  Scope5 : Scope
      settings: ActiveDisplayYMinimum=-0.125  ActiveDisplayYMaximum=1.125  DataLoggingVariableName=ScopeData10
  Torque_Limiter_Front : Subsystem
  Torque_Limiter_Rear : Subsystem
  state : Outport
  Out2 : Outport  Port=2
  Out3 : Outport  Port=3
  wires:
  omega_motor1/1 -> Anti_Shuffle_Damping_Rear/1(omega_motor)
  Mux2/1 -> Out3/1, Scope3/1
  Torque_Limiter_Rear/2(state) -> Scope5/1, Mux1/2
  Anti_Shuffle_Damping_Front/1(T_damp) -> Mux2/1
  Anti_Shuffle_Damping_Rear/1(T_damp) -> Mux2/2
  risk1/1 -> Torque_Limiter_Rear/2(risk)
  Torque_Limiter_Rear/1(Tlim) -> Scope1/2, Mux/2
  Mux1/1 -> Scope2/1
  Torque_Limiter_Front/1(Tlim) -> Scope1/1, Mux/1
  Torque_Limiter_Front/2(state) -> state/1, Mux1/1
  T_vcu1/1 -> Torque_Limiter_Rear/1(T_vcu)
  limit_ratio/1 -> Torque_Limiter_Front/4(limit_ratio)
  risk/1 -> Torque_Limiter_Front/2(risk)
  warn/1 -> Torque_Limiter_Front/3(warn)
  omega_motor/1 -> Anti_Shuffle_Damping_Front/1(omega_motor)
  limit_ratio1/1 -> Torque_Limiter_Rear/4(limit_ratio)
  Mux/1 -> Out2/1
  warn1/1 -> Torque_Limiter_Rear/3(warn)
  T_vcu/1 -> Torque_Limiter_Front/1(T_vcu)

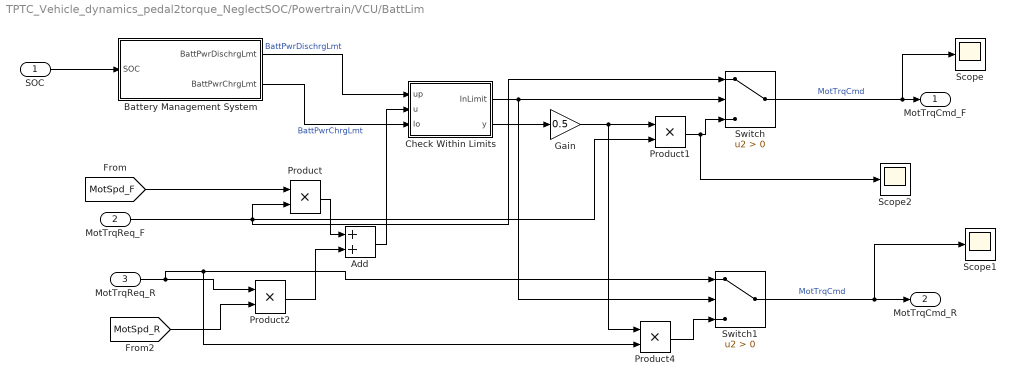
== system TPTC_Vehicle_dynamics_pedal2torque_NeglectSOC/Powertrain/VCU/BattLim ==
  SOC : Inport
  MotTrqReq_F : Inport  Port=2
  MotTrqReq_R : Inport  Port=3
  Add : Sum
  Battery Management System : Subsystem
  Check Within Limits : Subsystem
  Gain : Gain  Gain=0.5
  Product : Product
  Product1 : Product  Inputs=**
  Product2 : Product
  Product4 : Product  Inputs=**
  Scope : Scope
      settings: ActiveDisplayYMinimum=-1.92492538383E+6  ActiveDisplayYMaximum=1.732432845446E+7  DataLoggingVariableName=ScopeData15
  Scope1 : Scope
      settings: ActiveDisplayYMinimum=-1.92492538383E+6  ActiveDisplayYMaximum=1.732432845446E+7  DataLoggingVariableName=ScopeData16
  Scope2 : Scope
      settings: ActiveDisplayYMinimum=-1.92492538383E+6  ActiveDisplayYMaximum=1.732432845447E+7  DataLoggingVariableName=ScopeData17
  Switch : Switch  Criteria=u2 > Threshold  SaturateOnIntegerOverflow=off  InputSameDT=off
  Switch1 : Switch  Criteria=u2 > Threshold  SaturateOnIntegerOverflow=off  InputSameDT=off
  MotTrqCmd_F : Outport
  MotTrqCmd_R : Outport  Port=2
  wires:
  Check Within Limits/1(InLimit) -> Switch1/2, Switch/2
  MotTrqReq_F/1 -> Product1/2, Switch/1, Product/2
  Check Within Limits/2(y) -> Gain/1
  [MotSpd_F] -> Product/1
  Battery Management System/2(BattPwrChrgLmt) -> Check Within Limits/3(lo)  "BattPwrChrgLmt"
  Battery Management System/1(BattPwrDischrgLmt) -> Check Within Limits/1(up)  "BattPwrDischrgLmt"
  SOC/1 -> Battery Management System/1(SOC)
  Switch/1 -> Scope/1, MotTrqCmd_F/1  "MotTrqCmd"
  [MotSpd_R] -> Product2/2
  Product/1 -> Add/1
  Product2/1 -> Add/2
  Add/1 -> Check Within Limits/2(u)
  Switch1/1 -> Scope1/1, MotTrqCmd_R/1  "MotTrqCmd"
  MotTrqReq_R/1 -> Product4/2, Switch1/1, Product2/1
  Gain/1 -> Product4/1, Product1/1
  Product4/1 -> Switch1/3
  Product1/1 -> Scope2/1, Switch/3

== system TPTC_Vehicle_dynamics_pedal2torque_NeglectSOC/Powertrain/VCU/DecelPedaltoBrakePressReq ==
  DecelPedal : Inport
  Gain : Gain  Gain=5e6
  BrakePress : Outport
  wires:
  Gain/1 -> BrakePress/1
  DecelPedal/1 -> Gain/1

== system TPTC_Vehicle_dynamics_pedal2torque_NeglectSOC/Powertrain/03_MCU_TPTC_Controller/Torque_Limiter/Anti_Shuffle_Damping_Front ==
  omega_motor : Inport
  Damp_Limit : Saturate  UpperLimit=T_damp_lim  LowerLimit=-T_damp_lim
  HighPass : Sum  Inputs=+-
  LPF_omega : DiscreteTransferFcn  Numerator=[Ts_asr/tau_lpf_damp]  Denominator=[1 -(1-Ts_asr/tau_lpf_damp)]  SampleTime=Ts_asr
  Minus_Kd : Gain  Gain=-Kd_damp
  T_damp : Outport
  wires:
  omega_motor/1 -> LPF_omega/1, HighPass/1
  LPF_omega/1 -> HighPass/2
  HighPass/1 -> Minus_Kd/1
  Minus_Kd/1 -> Damp_Limit/1
  Damp_Limit/1 -> T_damp/1

== system TPTC_Vehicle_dynamics_pedal2torque_NeglectSOC/Powertrain/03_MCU_TPTC_Controller/Torque_Limiter/Anti_Shuffle_Damping_Rear ==
  omega_motor : Inport
  Damp_Limit : Saturate  UpperLimit=T_damp_lim  LowerLimit=-T_damp_lim
  HighPass : Sum  Inputs=+-
  LPF_omega : DiscreteTransferFcn  Numerator=[Ts_asr/tau_lpf_damp]  Denominator=[1 -(1-Ts_asr/tau_lpf_damp)]  SampleTime=Ts_asr
  Minus_Kd : Gain  Gain=-Kd_damp
  T_damp : Outport
  wires:
  omega_motor/1 -> LPF_omega/1, HighPass/1
  LPF_omega/1 -> HighPass/2
  HighPass/1 -> Minus_Kd/1
  Minus_Kd/1 -> Damp_Limit/1
  Damp_Limit/1 -> T_damp/1

== system TPTC_Vehicle_dynamics_pedal2torque_NeglectSOC/Powertrain/03_MCU_TPTC_Controller/Torque_Limiter/Torque_Limiter_Front ==
  T_vcu : Inport
  risk : Inport  Port=2
  warn : Inport  Port=3
  limit_ratio : Inport  Port=4
  Constant2 : Constant  Value=Ts_asr
  Fast_Down_Slow_Up_Limiter : MATLAB Function  TreatAsAtomicUnit=on  SystemSampleTime=Ts_asr
  Scope1 : Scope  NumInputPorts=2
      settings: ActiveDisplayYMinimum=-0.125  ActiveDisplayYMaximum=1.125  DataLoggingVariableName=ScopeData4
  Scope14 : Scope  NumInputPorts=2
      settings: ActiveDisplayYMinimum=-12.5  ActiveDisplayYMaximum=112.5  DataLoggingVariableName=ScopeData3
  Tlim : Outport
  state : Outport  Port=2
  wires:
  T_vcu/1 -> Fast_Down_Slow_Up_Limiter/1(T_req), Scope14/1
  risk/1 -> Scope1/1, Fast_Down_Slow_Up_Limiter/2(risk), Scope14/2
  warn/1 -> Scope1/2, Fast_Down_Slow_Up_Limiter/3(warn)
  Fast_Down_Slow_Up_Limiter/1(T_cmd_limited) -> Tlim/1
  Fast_Down_Slow_Up_Limiter/2(state) -> state/1
  Constant2/1 -> Fast_Down_Slow_Up_Limiter/6(Ts)
  limit_ratio/1 -> Fast_Down_Slow_Up_Limiter/5(Tlim_warn_rate), Fast_Down_Slow_Up_Limiter/4(limit_ratio)

== system TPTC_Vehicle_dynamics_pedal2torque_NeglectSOC/Powertrain/03_MCU_TPTC_Controller/Torque_Limiter/Torque_Limiter_Rear ==
  T_vcu : Inport
  risk : Inport  Port=2
  warn : Inport  Port=3
  limit_ratio : Inport  Port=4
  Constant2 : Constant  Value=Ts_asr
  Fast_Down_Slow_Up_Limiter : MATLAB Function  TreatAsAtomicUnit=on  SystemSampleTime=Ts_asr
  Scope : Scope  NumInputPorts=2
      settings: ActiveDisplayYMinimum=90  ActiveDisplayYMaximum=110  DataLoggingVariableName=ScopeData6
  Tlim : Outport
  state : Outport  Port=2
  wires:
  T_vcu/1 -> Scope/1, Fast_Down_Slow_Up_Limiter/1(T_req)
  risk/1 -> Fast_Down_Slow_Up_Limiter/2(risk)
  warn/1 -> Fast_Down_Slow_Up_Limiter/3(warn)
  Fast_Down_Slow_Up_Limiter/1(T_cmd_limited) -> Scope/2, Tlim/1
  Fast_Down_Slow_Up_Limiter/2(state) -> state/1
  limit_ratio/1 -> Fast_Down_Slow_Up_Limiter/5(Tlim_warn_rate), Fast_Down_Slow_Up_Limiter/4(limit_ratio)
  Constant2/1 -> Fast_Down_Slow_Up_Limiter/6(Ts)

== system TPTC_Vehicle_dynamics_pedal2torque_NeglectSOC/Powertrain/VCU/BattLim/Battery Management System ==
  note: Behaviorial BMS System. Limits battery charge / discharge power based on SOC.
      |
      | Charge/Discharge Limits and curves can be adjusted if using a larger battery pack
      | or motor power is changed.
  SOC : Inport
  ChrgLmt : Lookup_n-D  NumberOfTableDimensions=1  BreakpointsForDimension1=SOC_bpt  Table=ChrgLmt_bpt  ExtrapMethod=Clip  UseLastTableValue=on  InternalRulePriority=Speed  RndMeth=Simplest
  DischrgLmt : Lookup_n-D  NumberOfTableDimensions=1  BreakpointsForDimension1=SOC_bpt  Table=DischrgLmt_bpt  ExtrapMethod=Clip  UseLastTableValue=on  InternalRulePriority=Speed  RndMeth=Simplest
  MaxChrg : Constant  Value=BattChrgMax*0.8
  MaxDischrg : Constant  Value=BattDischrgMax*0.8
  Product : Product
  Product1 : Product
  BattPwrDischrgLmt : Outport  VectorParamsAs1DForOutWhenUnconnected=off
  BattPwrChrgLmt : Outport  Port=2  VectorParamsAs1DForOutWhenUnconnected=off
  wires:
  SOC/1 -> DischrgLmt/1, ChrgLmt/1
  MaxChrg/1 -> Product1/2
  MaxDischrg/1 -> Product/2
  Product/1 -> BattPwrDischrgLmt/1
  Product1/1 -> BattPwrChrgLmt/1
  ChrgLmt/1 -> Product1/1
  DischrgLmt/1 -> Product/1

== system TPTC_Vehicle_dynamics_pedal2torque_NeglectSOC/Powertrain/VCU/BattLim/Check Within Limits ==
  up : Inport
  u : Inport  Port=2
  lo : Inport  Port=3
  Compare To Zero : simulink/Logic and Bit Operations/Compare To Zero  relop=>=  OutDataTypeStr=boolean
  Compare To Zero1 : simulink/Logic and Bit Operations/Compare To Zero  relop=<=  OutDataTypeStr=boolean
  Logical Operator : Logic  AllPortsSameDT=off  OutDataTypeStr=boolean
  Saturation Dynamic1 : simulink/Discontinuities/Saturation Dynamic  OutMin=[]  OutMax=[]  OutDataTypeStr=Inherit: Same as second input  OutDataType=fixdt(1, 16)  OutScaling=2^-10  DoSatur=off
  Subtract : Sum  Inputs=+-
  Subtract1 : Sum  Inputs=-+
  InLimit : Outport  VectorParamsAs1DForOutWhenUnconnected=off
  y : Outport  Port=2  VectorParamsAs1DForOutWhenUnconnected=off
  wires:
  Saturation Dynamic1/1 -> y/1
  lo/1 -> Subtract1/2, Saturation Dynamic1/3
  up/1 -> Subtract/1, Saturation Dynamic1/1
  u/1 -> Subtract1/1, Subtract/2, Saturation Dynamic1/2
  Subtract/1 -> Compare To Zero/1
  Subtract1/1 -> Compare To Zero1/1
  Compare To Zero/1 -> Logical Operator/1
  Compare To Zero1/1 -> Logical Operator/2
  Logical Operator/1 -> InLimit/1

== matlab function TPTC_Vehicle_dynamics_pedal2torque_NeglectSOC/03_MCU_ASR_Controller1/Command_Merge_Front/Fast_Down_Slow_Up_Limiter ==
  data: T_vcu_f input; T_cmd_f output; T_vcu_r input; Tlim_f input; Tlim_r input; T_damp_f input; T_damp_r input; T_cmd_r output
function [T_cmd_f, T_cmd_r] = f(T_vcu_f, T_vcu_r, Tlim_f, Tlim_r, T_damp_f, T_damp_r)
%#codegen

% Front axle
T_base_f = min(T_vcu_f, Tlim_f);
T_tmp_f = T_base_f + T_damp_f;

if T_tmp_f > Tlim_f
    T_cmd_f = Tlim_f;
elseif T_tmp_f < 0
    T_cmd_f = 0;
else
    T_cmd_f = T_tmp_f;
end

% Rear axle
T_base_r = min(T_vcu_r, Tlim_r);
T_tmp_r = T_base_r + T_damp_r;

if T_tmp_r > Tlim_r
    T_cmd_r = Tlim_r;
elseif T_tmp_r < 0
    T_cmd_r = 0;
else
    T_cmd_r = T_tmp_r;
end

end

== matlab function TPTC_Vehicle_dynamics_pedal2torque_NeglectSOC/03_MCU_ASR_Controller1/Slip_Detector_Front/MATLAB Function ==
  data: Te input; risk output; warn output; alpha input; Tload input; omega input; Te_opp input; alpha_opp input; Tload_opp input; omega_opp input; T_active input; state output; alpha_thr input; Ts input; load_ratio output; follow_bad output; axis_diverge output; startup_guard output
function [risk,warn,state,load_ratio,follow_bad,axis_diverge,startup_guard] = f( ...
    Te,alpha,Tload,omega, ...
    Te_opp,alpha_opp,Tload_opp,omega_opp, ...
    T_active,alpha_thr,Ts)
%#codegen

% ============================================================
% MCU级 TCPC/ASR Slip Detector
%
% 核心判据：
% 1. Tload_est / Te 偏低
% 2. Te 增加时，Tload_est 不跟随增加
% 3. alpha 异常升高作为确认条件
%
% axis_diverge 只做诊断输出，不单独触发 warn/risk
%
% state:
%   0 Normal
%   1 Warning
%   2 Risk
% ============================================================

persistent risk_z warn_z
persistent Te_z Tload_z omega_z omega_opp_z
persistent active_cnt risk_enter_cnt warn_enter_cnt risk_exit_cnt warn_exit_cnt

if isempty(risk_z)
    risk_z = false;
    warn_z = false;

    Te_z = 0.0;
    Tload_z = 0.0;
    omega_z = 0.0;
    omega_opp_z = 0.0;

    active_cnt = 0.0;
    risk_enter_cnt = 0.0;
    warn_enter_cnt = 0.0;
    risk_exit_cnt = 0.0;
    warn_exit_cnt = 0.0;
end

% =========================
% 采样时间保护
% =========================
if Ts <= 0.0
    Ts_eff = 1e-3;
else
    Ts_eff = Ts;
end

% =========================
% 可标定参数
% =========================

% 负载比例阈值
k_load_risk = 0.72;
k_load_warn = 0.86;

% 跟随性阈值
k_follow_risk = 0.20;
k_follow_warn = 0.40;

% alpha 阈值
alpha_warn_gain = 0.65;
alpha_risk_gain = 1.00;

% 起步保护
startup_guard_time = 0.30;
startup_guard_steps = ceil(startup_guard_time / Ts_eff);

% 起步阶段只允许较强 risk
alpha_start_risk_gain = 1.40;
k_load_start_risk = 0.55;

% 进入确认时间
% risk 不要太慢，否则压不住滑移；warn 稍微确认
risk_enter_confirm_time = 0.005;  % 5 ms
warn_enter_confirm_time = 0.020;  % 20 ms

risk_enter_steps = ceil(risk_enter_confirm_time / Ts_eff);
warn_enter_steps = ceil(warn_enter_confirm_time / Ts_eff);

% 退出确认时间
risk_exit_confirm_time = 0.080;   % 80 ms，避免频繁退出
warn_exit_confirm_time = 0.050;   % 50 ms

risk_exit_steps = ceil(risk_exit_confirm_time / Ts_eff);
warn_exit_steps = ceil(warn_exit_confirm_time / Ts_eff);

% dTe 太小时不判断跟随性
dTe_min = max(0.02*T_active, 0.5);

% 前后轴分化诊断阈值
alpha_diff_thr = 0.80*alpha_thr;
omega_diff_thr = 5.0;
omega_diff_rate_thr = 50.0;

% =========================
% 有效驱动区
% =========================
active = (Te > T_active);

if active
    active_cnt = active_cnt + 1.0;
else
    active_cnt = 0.0;
end

startup_guard = active && (active_cnt <= startup_guard_steps);

% =========================
% 负载比例
% =========================
Te_eff = max(Te, 1.0);
load_ratio_raw = Tload / Te_eff;

if load_ratio_raw < 0.0
    load_ratio = 0.0;
elseif load_ratio_raw > 2.0
    load_ratio = 2.0;
else
    load_ratio = load_ratio_raw;
end

load_gap_risk = (load_ratio < k_load_risk);
load_gap_warn = (load_ratio < k_load_warn);

% =========================
% Tload 是否随 Te 增加
% =========================
dTe = Te - Te_z;
dTload = Tload - Tload_z;

torque_rising = (dTe > dTe_min);

follow_bad_risk = torque_rising && (dTload < k_follow_risk*dTe);
follow_bad_warn = torque_rising && (dTload < k_follow_warn*dTe);

follow_bad = follow_bad_risk;

% =========================
% alpha 异常
% =========================
alpha_risk = (alpha > alpha_risk_gain*alpha_thr);
alpha_warn = (alpha > alpha_warn_gain*alpha_thr);

% =========================
% 前后轴分化，仅诊断
% =========================
omega_diff = omega - omega_opp;
omega_diff_z = omega_z - omega_opp_z;
d_omega_diff = (omega_diff - omega_diff_z) / Ts_eff;

alpha_diverge = (alpha > alpha_opp + alpha_diff_thr) && alpha_warn;

omega_diverge = (~startup_guard) && ...
                (omega_diff > omega_diff_thr) && ...
                (d_omega_diff > omega_diff_rate_thr);

axis_diverge = alpha_diverge || omega_diverge;

% =========================
% 原始进入判据
% =========================
if startup_guard

    % 起步保护阶段：
    % 不允许 warn，只允许强 risk
    warn_enter_raw = false;

    risk_enter_raw = active && ...
                     (alpha > alpha_start_risk_gain*alpha_thr) && ...
                     ((load_ratio < k_load_start_risk) || follow_bad_risk);

else

    % 正常阶段：
    % axis_diverge 不直接触发
    risk_enter_raw = active && ...
                     alpha_risk && ...
                     (load_gap_risk || follow_bad_risk);

    warn_enter_raw = active && ...
                     alpha_warn && ...
                     (load_gap_warn || follow_bad_warn);
end

% =========================
% 进入确认
% =========================
if risk_enter_raw
    risk_enter_cnt = risk_enter_cnt + 1.0;
else
    risk_enter_cnt = 0.0;
end

if warn_enter_raw
    warn_enter_cnt = warn_enter_cnt + 1.0;
else
    warn_enter_cnt = 0.0;
end

risk_enter = (risk_enter_cnt >= risk_enter_steps);
warn_enter = (warn_enter_cnt >= warn_enter_steps);

% =========================
% 退出判据
% =========================
risk_exit_raw = (~active) || ...
                ( ...
                  (alpha < 0.45*alpha_thr) && ...
                  (load_ratio > 0.88) && ...
                  (~follow_bad_warn) ...
                );

warn_exit_raw = (~active) || ...
                ( ...
                  (alpha < 0.35*alpha_thr) && ...
                  (load_ratio > 0.96) && ...
                  (~follow_bad_warn) ...
                );

if risk_exit_raw
    risk_exit_cnt = risk_exit_cnt + 1.0;
else
    risk_exit_cnt = 0.0;
end

if warn_exit_raw
    warn_exit_cnt = warn_exit_cnt + 1.0;
else
    warn_exit_cnt = 0.0;
end

risk_exit = (risk_exit_cnt >= risk_exit_steps);
warn_exit = (warn_exit_cnt >= warn_exit_steps);

% =========================
% risk 滞回
% =========================
if risk_z
    if risk_exit
        risk_z = false;
        risk_exit_cnt = 0.0;
    end
else
    if risk_enter
        risk_z = true;
        risk_enter_cnt = 0.0;
    end
end

% =========================
% warn 滞回
% =========================
if risk_z
    warn_z = false;
    warn_exit_cnt = 0.0;
else
    if warn_z
        if warn_exit
            warn_z = false;
            warn_exit_cnt = 0.0;
        end
    else
        if warn_enter
            warn_z = true;
            warn_enter_cnt = 0.0;
        end
    end
end

% =========================
% 输出
% =========================
risk = risk_z;
warn = warn_z;

if risk_z
    state = 2.0;
elseif warn_z
    state = 1.0;
else
    state = 0.0;
end

% =========================
% 更新历史量
% =========================
Te_z = Te;
Tload_z = Tload;
omega_z = omega;
omega_opp_z = omega_opp;

end
